simulink model "buenoensamy6"  (R2013a)
settings: Solver=ode45  StartTime=0.0  StopTime=80  FixedStep=1  RelTol=1e-3
values from neighbouring files (symbols this model uses):
  g = 9.81    [miosinlazoalgebraico1.m]    (also in proyectoy6.m)
  I1 = .004    (= 0.004)    [miosinlazoalgebraico1.m]    (also in proyectoy6.m = 0.0004)
  lc2 = .062    (= 0.062)    [miosinlazoalgebraico1.m]    (also in proyectoy6.m = 0.09)
  m2 = .7175    (= 0.7175)    [miosinlazoalgebraico1.m]    (also in proyectoy6.m = 0.0928)
  theta2 = (m2*lc2*lc2)+I2    (= 0.00775807)    [miosinlazoalgebraico1.m]    (also in proyectoy6.m = 0.00125168)
  theta3 = (m2*l1*lc2)    (= 0.008897)    [miosinlazoalgebraico1.m]    (also in proyectoy6.m = 0.00091872)
  theta4 = (m1*lc1)+(m2*l1)    (= 0.495148)    [miosinlazoalgebraico1.m]    (also in proyectoy6.m = 0.014993)
  theta5 = (m2*lc2)    (= 0.044485)    [miosinlazoalgebraico1.m]    (also in proyectoy6.m = 0.008352)
  theta6 = (m1*lc1*lc1)+(m2*l1*l1)    (= 0.09375488)    [miosinlazoalgebraico1.m]    (also in proyectoy6.m = 0.001386055)
undefined symbols (not defined in the file or in its folder): base, buenoensam, Pieza2, Pieza3, RootGround, RootPart
libraries: mblibv1 x14
settings Model: Creator=Daniel  LastModifiedBy=Daniel
settings SolverCC: MaxConsecutiveZCs=100000  ZeroCrossAlgorithm=Adaptive
settings SimMechanicsCC: VisOnUpdateDiagram=on  VisDuringSimulation=on

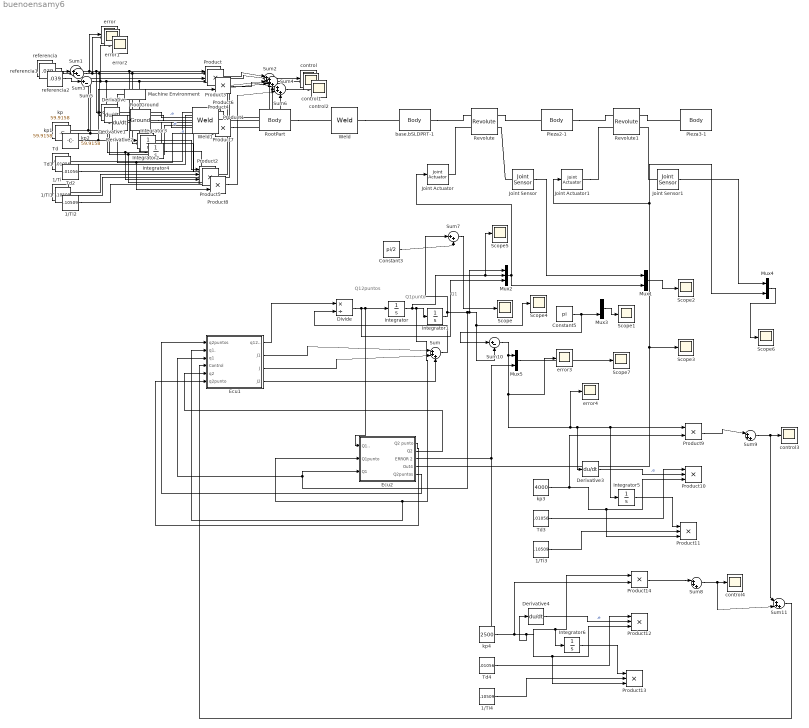
== system buenoensamy6 ==
  note: Q1
  note: Q1punto
  note: Q12puntos
  1/Ti{,1..4} (5 alike) : Constant  Value=.10509
  Constant3 : Constant  Value=pi/2
  Constant5 : Constant  Value=pi
  Derivative{,1..4} (5 alike) : Derivative
  Divide : Product  Inputs=*/
  Ecu1 : Subsystem
  Ecu2 : Subsystem
  Integrator{,2..6} (6 alike) : Integrator
  Integrator1 : Integrator  InitialCondition=pi/2  IgnoreLimit=on
  Joint Actuator : mblibv1/Sensors &  Actuators/Joint Actuator  UpdateFromCAD=off  PhysicalDomain=Mechanical  PortType=blob  ActuationStyle=Motion  AngleUnits=rad  ArcVelocityUnits=rad/s  ArcAccelerationUnits=rad/s^2  CoordPositionUnits=m  VelocityUnits=m/s  AccelerationUnits=m/s^2  ForceUnits=N  TorqueUnits=N*m  ActiveIO=on  Width=3  DialogClass=MechanicalActuatorBlock  Primitive=R1  ReferenceFrame=Absolute (World)
  Joint Actuator1 : mblibv1/Sensors &  Actuators/Joint Actuator  UpdateFromCAD=off  PhysicalDomain=Mechanical  PortType=blob  ActuationStyle=Motion  AngleUnits=rad  ArcVelocityUnits=rpm  ArcAccelerationUnits=rad/s^2  CoordPositionUnits=m  VelocityUnits=m/s  AccelerationUnits=m/s^2  ForceUnits=N  TorqueUnits=N*m  ActiveIO=on  Width=3  DialogClass=MechanicalActuatorBlock  Primitive=R1  ReferenceFrame=Absolute (World)
  Joint Sensor : mblibv1/Sensors &  Actuators/Joint Sensor  UpdateFromCAD=off  PhysicalDomain=Mechanical  PortType=blob  Muxed=on  Pose=off  Angle=on  AngleUnits=rad  ArcVelocity=off  ArcVelocityUnits=deg/s  ArcAcceleration=off  ArcAccelerationUnits=deg/s^2  CoordPosition=on  CoordPositionUnits=m  Velocity=off  VelocityUnits=m/s  Acceleration=off  AccelerationUnits=m/s^2  Quaternion=on  QuaternionDT=off  QuaternionDDT=off  QuaternionUnits=off  OutputVector=[1]  ActiveIO=on  Width=1  DialogClass=MechanicalSensorBlock  Primitive=R1  Force=off  ForceUnits=N  Torque=off  TorqueUnits=N*m  ReferenceFrame=Absolute (World)  ReactionSensedSide=Base  ReactionReferenceFrame=Absolute (World)  ReactionForce=off  ReactionForceUnits=N  ReactionMoment=off  ReactionMomentUnits=N*m
  Joint Sensor1 : mblibv1/Sensors &  Actuators/Joint Sensor  UpdateFromCAD=off  PhysicalDomain=Mechanical  PortType=blob  Muxed=on  Pose=off  Angle=on  AngleUnits=deg  ArcVelocity=off  ArcVelocityUnits=deg/s  ArcAcceleration=off  ArcAccelerationUnits=deg/s^2  CoordPosition=on  CoordPositionUnits=m  Velocity=off  VelocityUnits=m/s  Acceleration=off  AccelerationUnits=m/s^2  Quaternion=on  QuaternionDT=off  QuaternionDDT=off  QuaternionUnits=off  OutputVector=[1]  ActiveIO=on  Width=1  DialogClass=MechanicalSensorBlock  Primitive=R1  Force=off  ForceUnits=N  Torque=off  TorqueUnits=N-m  ReferenceFrame=Absolute (World)  ReactionSensedSide=Base  ReactionReferenceFrame=Absolute (World)  ReactionForce=off  ReactionForceUnits=N  ReactionMoment=off  ReactionMomentUnits=N-m
  Machine Environment : mblibv1/Bodies/Machine Environment  PortType=env  PhysicalDomain=Mechanical  DialogTemplateClass=MECH.MachineEnvironment  SyncWhenCopied=off  Gravity=[0 -9.81 0]  GravityUnits=m/s^2  GravityAsSignal=off  Dimensionality=Auto-detect  AnalysisType=Forward dynamics  LinearAssemblyTolerance=1e-3  LinearAssemblyToleranceUnits=m  AngularAssemblyTolerance=1e-3  AngularAssemblyToleranceUnits=rad  ConstraintSolverType=Stabilizing  ConstraintRelTolerance=1e-4  ConstraintAbsTolerance=1e-4  UseRobustSingularityHandling=off  RedundancyAnalysisToleranceType=Automatically select tolerance  RedundancyAnalysisTolerance=1e-14  StatePerturbationType=Fixed  PerturbationSize=1e-5  VisualizeMachine=on  BodyVisualizationType=Use model default body geometries  BodyColorSelMode=Use model default  DefaultBodyColor=[1 0 0]
  Mux{1,3..5} (4 alike) : Mux  Inputs=2
  Mux2 : Mux  Inputs=3
  Pieza2-1 : mblibv1/Bodies/Body  LConnTagsString=CS2  RConnTagsString=CS3  UpdateFromCAD=on  PMImportedID=Pieza2-1  DialogClass=MechanicalBodyBlock  Mass=0.734204  MassUnits=kg  InertiaUnits=kg*m^2  Inertia=[0.000264247,2.83059e-10,-6.28102e-08;2.83059e-10,0.0127231,5.8833e-11;-6.28102e-08,5.8833e-11,0.0126365]  Shape=Cylinder  ShapeDims=[1 1]  ShapeUnits=m  ShapeUse=false  Density=1  DensityUnits=kg/m^3  DensityUse=false  GraphicsMode=GFXFILE  GraphicsFileName=buenoensam - Pieza2-1.STL  BodyColorSelMode=COLORPALETTE  BodyColor=[1;1;0]  AttachedToCS=CS1  CG=Right$CG$[-0.0307943 -0.183465 0.38735]$WORLD$WORLD$m$[0.0349053 0 -0.999391;-0.999391 0 -0.0349053;0 1 0]$3x3 Transform$rad$WORLD$false$Pieza2-1::CG(AUTOGEN)  WorkingFrames=Right$CS1$[-0.0615922 -0.0278733 0.3683]$WORLD$WORLD$m$[0.0349053 0 -0.999391;-0.999391 0 -0.0349053;0 1 0]$3x3 Transform$rad$WORLD$false$Pieza2-1::CS1(AUTOGEN)#Left$CS2$[-0.0384461 0.0361919 0.3683]$WORLD$WORLD$m$[1 0 0;0 1 0;0 0 1]$3x3 Transform$rad$WORLD$true$Pieza2-1:-:base.bSLDPRT-1::Pieza2-1(AUTOGEN)#Right$CS3$[-0.0234804 -0.394088 0.3683]$WORLD$WORLD$m$[1 0 0;0 1 0;0 0 1]$3x3 Transform$rad$WORLD$true$Pieza2-1:-:Pieza3-1::Pieza2-1(AUTOGEN)  CGPos=[-0.0307943 -0.183465 0.38735]  CGRot=[0.0349053 0 -0.999391;-0.999391 0 -0.0349053;0 1 0]  CS0Pos=[]  CS0Rot=[]  CS1Pos=[-0.0615922 -0.0278733 0.3683]  CS1Rot=[0.0349053 0 -0.999391;-0.999391 0 -0.0349053;0 1 0]  CS2Pos=[-0.0384461 0.0361919 0.3683]  CS2Rot=[1 0 0;0 1 0;0 0 1]  CS3Pos=[-0.0234804 -0.394088 0.3683]  CS3Rot=[1 0 0;0 1 0;0 0 1]  CS4Pos=[]  CS4Rot=[]  CS5Pos=[]  CS5Rot=[]  CS6Pos=[]  CS6Rot=[]  CS7Pos=[]  CS7Rot=[]  CS8Pos=[]  CS8Rot=[]  CS9Pos=[]  CS9Rot=[]  CS10Pos=[]  CS10Rot=[]  CS11Pos=[]  CS11Rot=[]  CS12Pos=[]  CS12Rot=[]  CS13Pos=[]  CS13Rot=[]  CS14Pos=[]  CS14Rot=[]  CS15Pos=[]  CS15Rot=[]  CS16Pos=[]  CS16Rot=[]  CS17Pos=[]  CS17Rot=[]  CS18Pos=[]  CS18Rot=[]  CS19Pos=[]  CS19Rot=[]  CS20Pos=[]  CS20Rot=[]
  Pieza3-1 : mblibv1/Bodies/Body  LConnTagsString=CS2  UpdateFromCAD=on  PMImportedID=Pieza3-1  DialogClass=MechanicalBodyBlock  Mass=0.784305  MassUnits=kg  InertiaUnits=kg*m^2  Inertia=[0.000374519,0.000457935,-7.77784e-07;0.000457935,0.0141418,4.97542e-08;-7.77784e-07,4.97542e-08,0.0141799]  Shape=Cylinder  ShapeDims=[1 1]  ShapeUnits=m  ShapeUse=false  Density=1  DensityUnits=kg/m^3  DensityUse=false  GraphicsMode=GFXFILE  GraphicsFileName=buenoensam - Pieza3-1.STL  BodyColorSelMode=COLORPALETTE  BodyColor=[0;1;1]  AttachedToCS=CS1  CG=Right$CG$[-0.0137132 -0.5717 0.352532]$WORLD$WORLD$m$[0.0550174 0 -0.998485;-0.998485 0 -0.0550174;0 1 0]$3x3 Transform$rad$WORLD$false$Pieza3-1::CG(AUTOGEN)  WorkingFrames=Right$CS1$[-0.0453321 -0.458607 0.3302]$WORLD$WORLD$m$[0.0550174 0 -0.998485;-0.998485 0 -0.0550174;0 1 0]$3x3 Transform$rad$WORLD$false$Pieza3-1::CS1(AUTOGEN)#Left$CS2$[-0.0234804 -0.394088 0.3683]$WORLD$WORLD$m$[1 0 0;0 1 0;0 0 1]$3x3 Transform$rad$WORLD$true$Pieza2-1:-:Pieza3-1::Pieza3-1(AUTOGEN)  CGPos=[-0.0137132 -0.5717 0.352532]  CGRot=[0.0550174 0 -0.998485;-0.998485 0 -0.0550174;0 1 0]  CS0Pos=[]  CS0Rot=[]  CS1Pos=[-0.0453321 -0.458607 0.3302]  CS1Rot=[0.0550174 0 -0.998485;-0.998485 0 -0.0550174;0 1 0]  CS2Pos=[-0.0234804 -0.394088 0.3683]  CS2Rot=[1 0 0;0 1 0;0 0 1]  CS3Pos=[]  CS3Rot=[]  CS4Pos=[]  CS4Rot=[]  CS5Pos=[]  CS5Rot=[]  CS6Pos=[]  CS6Rot=[]  CS7Pos=[]  CS7Rot=[]  CS8Pos=[]  CS8Rot=[]  CS9Pos=[]  CS9Rot=[]  CS10Pos=[]  CS10Rot=[]  CS11Pos=[]  CS11Rot=[]  CS12Pos=[]  CS12Rot=[]  CS13Pos=[]  CS13Rot=[]  CS14Pos=[]  CS14Rot=[]  CS15Pos=[]  CS15Rot=[]  CS16Pos=[]  CS16Rot=[]  CS17Pos=[]  CS17Rot=[]  CS18Pos=[]  CS18Rot=[]  CS19Pos=[]  CS19Rot=[]  CS20Pos=[]  CS20Rot=[]
  Product{,3,6,9,14} (5 alike) : Product
  Product{1..2,4..5,7..8,10..13} (10 alike) : Product  Inputs=3
  Revolute : mblibv1/Joints/Revolute  LConnTagsString=__newl0|SA1  RConnTagsString=__newr0|SA1  UpdateFromCAD=on  PMImportedID=Pieza2-1:-:base.bSLDPRT-1  NumSAPorts=2  CutJoint=off  MarkAsCut=off  Primitives=prismatic  PrimitiveProps=R1$World$[0,0,-1]$revolute  DialogClass=JointBlock  R1Axis=[0,0,-1]
  Revolute1 : mblibv1/Joints/Revolute  LConnTagsString=__newl0|SA1  RConnTagsString=__newr0|SA1  UpdateFromCAD=on  PMImportedID=Pieza2-1:-:Pieza3-1  NumSAPorts=2  CutJoint=off  MarkAsCut=off  Primitives=prismatic  PrimitiveProps=R1$World$[0,0,1]$revolute  DialogClass=JointBlock  R1Axis=[0,0,1]
  RootGround : mblibv1/Bodies/Ground  UpdateFromCAD=on  PMImportedID=RootGround  LeftPortType=env  RightPortType=workingframe  PhysicalDomain=Mechanical  DialogClass=GroundBlock  CoordPosition=[-0.0313325,-0.14828,0.31783]  CoordPositionUnits=m  StateVectorMgrId=-1  MachineId=[0 0]  ShowEnvPort=on
  RootPart : mblibv1/Bodies/Body  LConnTagsString=CS3  RConnTagsString=CS2  UpdateFromCAD=on  PMImportedID=buenoensam/RootPart  DialogClass=MechanicalBodyBlock  Mass=0  MassUnits=kg  InertiaUnits=kg*m^2  Inertia=[0,0,0;0,0,0;0,0,0]  Shape=Cylinder  ShapeDims=[1 1]  ShapeUnits=m  ShapeUse=false  Density=1  DensityUnits=kg/m^3  DensityUse=false  GraphicsMode=MACHINE_DEFAULT  BodyColorSelMode=MACHINE_DEFAULT  BodyColor=[1;0;0]  AttachedToCS=CS1  CG=Right$CG$[-0.0313325 -0.14828 0.31783]$WORLD$WORLD$m$[1 0 0;0 1 0;0 0 1]$3x3 Transform$rad$WORLD$false$buenoensam/RootPart::CG(AUTOGEN)  WorkingFrames=Right$CS1$[0 0 0]$WORLD$WORLD$m$[1 0 0;0 1 0;0 0 1]$3x3 Transform$rad$WORLD$false$buenoensam/RootPart::CS1(AUTOGEN)#Right$CS2$[-0.0384461 0.0308496 0.278664]$WORLD$WORLD$m$[1 0 0;0 1 0;0 0 1]$3x3 Transform$rad$WORLD$true$base.bSLDPRT-1:-:buenoensam/RootPart::buenoensam/RootPart(AUTOGEN)#Left$CS3$[-0.0313325 -0.14828 0.31783]$WORLD$WORLD$m$[1 0 0;0 1 0;0 0 1]$3x3 Transform$rad$WORLD$true$RootGround:-:buenoensam/RootPart::buenoensam/RootPart(AUTOGEN)  CGPos=[-0.0313325 -0.14828 0.31783]  CGRot=[1 0 0;0 1 0;0 0 1]  CS0Pos=[]  CS0Rot=[]  CS1Pos=[0 0 0]  CS1Rot=[1 0 0;0 1 0;0 0 1]  CS2Pos=[-0.0384461 0.0308496 0.278664]  CS2Rot=[1 0 0;0 1 0;0 0 1]  CS3Pos=[-0.0313325 -0.14828 0.31783]  CS3Rot=[1 0 0;0 1 0;0 0 1]  CS4Pos=[]  CS4Rot=[]  CS5Pos=[]  CS5Rot=[]  CS6Pos=[]  CS6Rot=[]  CS7Pos=[]  CS7Rot=[]  CS8Pos=[]  CS8Rot=[]  CS9Pos=[]  CS9Rot=[]  CS10Pos=[]  CS10Rot=[]  CS11Pos=[]  CS11Rot=[]  CS12Pos=[]  CS12Rot=[]  CS13Pos=[]  CS13Rot=[]  CS14Pos=[]  CS14Rot=[]  CS15Pos=[]  CS15Rot=[]  CS16Pos=[]  CS16Rot=[]  CS17Pos=[]  CS17Rot=[]  CS18Pos=[]  CS18Rot=[]  CS19Pos=[]  CS19Rot=[]  CS20Pos=[]  CS20Rot=[]
  Scope{,1..7} (8 alike) : Scope
      Scope settings: TimeRange=15  YMin=1.5e-07  YMax=1.1e-06
      Scope1 settings: TimeRange=15  YMin=1.5707963267948  YMax=1.5707963267956  SaveName=ScopeData5
      Scope2 settings: YMin=-1.2e+17  YMax=7e+16  SaveName=ScopeData2
      Scope3 settings: YMin=-0.7  YMax=0.1  SaveName=ScopeData3
      Scope4 settings: TimeRange=15  YMin=404  YMax=424
      Scope5 settings: TimeRange=40  YMin=-0.675  YMax=-0.225  SaveName=ScopeData6
      Scope6 settings: YMin=-1.2e+17  YMax=7e+16  SaveName=ScopeData7
      Scope7 settings: YMin=-0.7  YMax=0.1  SaveName=ScopeData8
  Sum{,2,4,6,8..9,11} (7 alike) : Sum  Inputs=|+++
  Sum{1,3,5,10} (4 alike) : Sum  Inputs=|+-
  Sum7 : Sum  Inputs=|++
  Td{,1..4} (5 alike) : Constant  Value=.01056
  Weld : mblibv1/Joints/Weld  LConnTagsString=__newl0  RConnTagsString=__newr0  UpdateFromCAD=on  PMImportedID=base.bSLDPRT-1:-:buenoensam/RootPart  NumSAPorts=0  CutJoint=off  MarkAsCut=off  Primitives=weld  PrimitiveProps=W$WORLD$[0.57735,0.57735,0.57735]$weld  DialogClass=JointBlock  WAxis=[0.57735,0.57735,0.57735]
  Weld1 : mblibv1/Joints/Weld  LConnTagsString=__newl0  RConnTagsString=__newr0  UpdateFromCAD=on  PMImportedID=RootGround:-:buenoensam/RootPart  NumSAPorts=0  CutJoint=off  MarkAsCut=off  Primitives=weld  PrimitiveProps=W$WORLD$[0.57735,0.57735,0.57735]$weld  DialogClass=JointBlock  WAxis=[0.57735,0.57735,0.57735]
  base.bSLDPRT-1 : mblibv1/Bodies/Body  LConnTagsString=CS2  RConnTagsString=CS3  UpdateFromCAD=on  PMImportedID=base.bSLDPRT-1  DialogClass=MechanicalBodyBlock  Mass=1.99812  MassUnits=kg  InertiaUnits=kg*m^2  Inertia=[0.0110019,0,0;0,0.0129359,-0.000127709;0,-0.000127709,0.00347297]  Shape=Cylinder  ShapeDims=[1 1]  ShapeUnits=m  ShapeUse=false  Density=1  DensityUnits=kg/m^3  DensityUse=false  GraphicsMode=GFXFILE  GraphicsFileName=buenoensam - base.bSLDPRT-1.STL  BodyColorSelMode=COLORPALETTE  BodyColor=[0;0;1]  AttachedToCS=CS1  CG=Right$CG$[-0.0384461 0.0308496 0.278664]$WORLD$WORLD$m$[1 0 0;0 1 0;0 0 1]$3x3 Transform$rad$WORLD$false$base.bSLDPRT-1::CG(AUTOGEN)  WorkingFrames=Right$CS1$[-0.0384461 -0.00190807 0.1651]$WORLD$WORLD$m$[1 0 0;0 1 0;0 0 1]$3x3 Transform$rad$WORLD$false$base.bSLDPRT-1::CS1(AUTOGEN)#Left$CS2$[-0.0384461 0.0308496 0.278664]$WORLD$WORLD$m$[1 0 0;0 1 0;0 0 1]$3x3 Transform$rad$WORLD$true$base.bSLDPRT-1:-:buenoensam/RootPart::base.bSLDPRT-1(AUTOGEN)#Right$CS3$[-0.0384461 0.0361919 0.3683]$WORLD$WORLD$m$[1 0 0;0 1 0;0 0 1]$3x3 Transform$rad$WORLD$true$Pieza2-1:-:base.bSLDPRT-1::base.bSLDPRT-1(AUTOGEN)  CGPos=[-0.0384461 0.0308496 0.278664]  CGRot=[1 0 0;0 1 0;0 0 1]  CS0Pos=[]  CS0Rot=[]  CS1Pos=[-0.0384461 -0.00190807 0.1651]  CS1Rot=[1 0 0;0 1 0;0 0 1]  CS2Pos=[-0.0384461 0.0308496 0.278664]  CS2Rot=[1 0 0;0 1 0;0 0 1]  CS3Pos=[-0.0384461 0.0361919 0.3683]  CS3Rot=[1 0 0;0 1 0;0 0 1]  CS4Pos=[]  CS4Rot=[]  CS5Pos=[]  CS5Rot=[]  CS6Pos=[]  CS6Rot=[]  CS7Pos=[]  CS7Rot=[]  CS8Pos=[]  CS8Rot=[]  CS9Pos=[]  CS9Rot=[]  CS10Pos=[]  CS10Rot=[]  CS11Pos=[]  CS11Rot=[]  CS12Pos=[]  CS12Rot=[]  CS13Pos=[]  CS13Rot=[]  CS14Pos=[]  CS14Rot=[]  CS15Pos=[]  CS15Rot=[]  CS16Pos=[]  CS16Rot=[]  CS17Pos=[]  CS17Rot=[]  CS18Pos=[]  CS18Rot=[]  CS19Pos=[]  CS19Rot=[]  CS20Pos=[]  CS20Rot=[]
  control{,1..4} (5 alike) : Scope
      control settings: YMin=77.5  YMax=84  SaveName=ScopeData4
      control1 settings: YMin=77.5  YMax=84  SaveName=ScopeData10
      control2 settings: YMin=77.5  YMax=84  SaveName=ScopeData12
      control3 settings: YMin=77.5  YMax=84  SaveName=ScopeData14
      control4 settings: YMin=77.5  YMax=84  SaveName=ScopeData17
  error{,1..4} (5 alike) : Scope
      error settings: YMin=-0.003  YMax=0.014  SaveName=ScopeData9
      error1 settings: YMin=-0.003  YMax=0.014  SaveName=ScopeData11
      error2 settings: YMin=-0.003  YMax=0.014  SaveName=ScopeData13
      error3 settings: YMin=-0.003  YMax=0.014  SaveName=ScopeData15
      error4 settings: YMin=-0.003  YMax=0.014  SaveName=ScopeData16
  kp : Constant  Value=59.9158
  kp1 : Constant  Value=59.9158
  kp2 : Constant  Value=59.9158
  kp3 : Constant  Value=4000
  kp4 : Constant  Value=2500
  referencia : Constant  Value=.039
  referencia1 : Constant  Value=.039
  referencia2 : Constant  Value=.039
  wires:
  Divide/1 -> Mux2/3, Ecu2/1(Q1..), Integrator/1
  Integrator/1 -> Scope5/1, Mux2/2, Integrator1/1, Ecu2/2(Q1punto), Ecu1/2(q1.)
  Sum/1 -> Divide/2
  Mux2/1 -> Joint Actuator/1, Mux1/2
  Joint Sensor/1 -> Mux1/1
  Mux1/1 -> Scope2/1
  Joint Sensor1/1 -> Mux4/1
  Constant3/1 -> Sum7/2
  Sum7/1 -> Scope/1
  Constant5/1 -> Sum10/1, Mux3/2
  Ecu2/2(Q2) -> Ecu1/5("q2 ")
  Ecu2/4(Out4) -> Scope3/1, Mux4/2, Joint Actuator1/1
  Ecu2/1(Q2 punto) -> Ecu1/6(q2punto)
  Ecu1/1(q12..) -> Divide/1
  Ecu1/2(J1) -> Sum/1
  Ecu1/3(J) -> Sum/2
  Ecu1/4(J2) -> Sum/3
  Mux3/1 -> Scope1/1
  Mux4/1 -> Scope6/1
  Ecu2/5(Q2puntos) -> Ecu1/1(q2puntos)
  Mux5/1 -> Scope7/1
  Integrator1/1 -> Sum7/1, Ecu2/3("Q1 "), Ecu1/3(q1), Mux2/1, Scope4/1, Sum10/2
  referencia/1 -> Sum1/1
  Sum1/1 -> error/1, Derivative/1, Product/1, Integrator2/1
  kp/1 -> Product/2, Product2/3, Product1/3
  Product/1 -> Sum2/1
  ? -> Sum1/2
  1/Ti/1 -> Product2/2
  Product1/1 -> Sum2/3
  Sum2/1 -> control/1
  Derivative/1 -> Product1/2  ".e"
  Td/1 -> Product1/1
  Product2/1 -> Sum2/2
  Integrator2/1 -> Product2/1
  referencia1/1 -> Sum3/1
  Sum3/1 -> error1/1, Derivative1/1, Product3/1, Integrator3/1
  kp1/1 -> Product3/2, Product5/3, Product4/3
  Product3/1 -> Sum4/1
  ? -> Sum3/2
  1/Ti1/1 -> Product5/2
  Product4/1 -> Sum4/3
  Sum4/1 -> control1/1
  Derivative1/1 -> Product4/2  ".e"
  Td1/1 -> Product4/1
  Product5/1 -> Sum4/2
  Integrator3/1 -> Product5/1
  referencia2/1 -> Sum5/1
  Sum5/1 -> error2/1, Derivative2/1, Product6/1, Integrator4/1
  kp2/1 -> Product6/2, Product8/3, Product7/3
  Product6/1 -> Sum6/1
  ? -> Sum5/2
  1/Ti2/1 -> Product8/2
  Product7/1 -> Sum6/3
  Sum6/1 -> control2/1
  Derivative2/1 -> Product7/2  ".e"
  Td2/1 -> Product7/1
  Product8/1 -> Sum6/2
  Integrator4/1 -> Product8/1
  Sum10/1 -> Integrator5/1, Product9/1, Derivative3/1, error4/1, error3/1, Mux5/1
  kp3/1 -> Product10/3, Product11/3, Product9/2
  Product9/1 -> Sum9/1
  1/Ti3/1 -> Product11/2
  Sum9/1 -> Sum11/1, control3/1
  Derivative3/1 -> Product10/2  ".e"
  Td3/1 -> Product10/1
  Integrator5/1 -> Product11/1
  Ecu2/3(ERROR 2) -> Mux5/2, Product14/1, Integrator6/1, Derivative4/1
  kp4/1 -> Product14/2, Product13/3, Product12/3
  1/Ti4/1 -> Product13/2
  Sum8/1 -> Sum11/2, control4/1
  Derivative4/1 -> Product12/2  ".e"
  Td4/1 -> Product12/1
  Integrator6/1 -> Product13/1
  Product14/1 -> Sum8/1
  Sum11/1 -> Ecu1/4("Control ")
  connections:
  RootPart/RConn1 -- Weld/LConn1
  Weld/RConn1 -- base.bSLDPRT-1/LConn1
  base.bSLDPRT-1/RConn1 -- Revolute/LConn1
  Revolute/RConn1 -- Pieza2-1/LConn1
  Pieza2-1/RConn1 -- Revolute1/LConn1
  Revolute1/RConn1 -- Pieza3-1/LConn1
  RootGround/RConn1 -- Weld1/LConn1
  Weld1/RConn1 -- RootPart/LConn1
  RootGround/LConn1 -- Machine Environment/RConn1
  Joint Actuator/RConn1 -- Revolute/LConn2
  Joint Sensor/LConn1 -- Revolute/RConn2
  Joint Actuator1/RConn1 -- Revolute1/LConn2
  Joint Sensor1/LConn1 -- Revolute1/RConn2

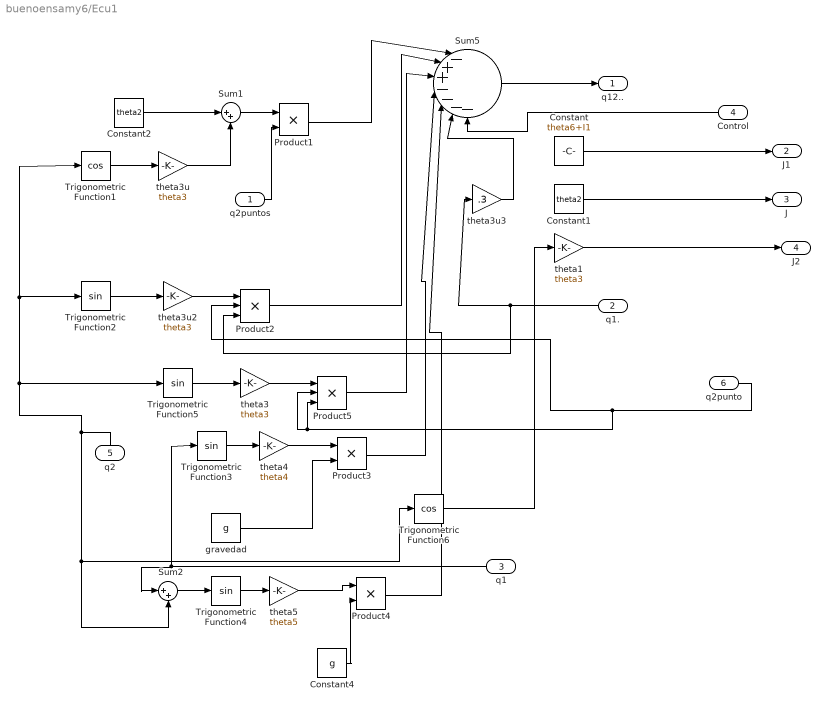
== system buenoensamy6/Ecu1 ==
  q2puntos : Inport
  q1. : Inport  Port=2
  q1 : Inport  Port=3
  "Control " : Inport  Port=4
  "q2 " : Inport  Port=5
  q2punto : Inport  Port=6
  Constant : Constant  Value=theta6+I1
  Constant1 : Constant  Value=theta2
  Constant2 : Constant  Value=theta2
  Constant4 : Constant  Value=g
  Product1 : Product
  Product2 : Product  Inputs=3
  Product3 : Product
  Product4 : Product
  Product5 : Product  Inputs=3
  Sum1 : Sum  Inputs=|++
  Sum2 : Sum  Inputs=|++
  Sum5 : Sum  Inputs=|-++----
  Trigonometric Function1 : Trigonometry  Operator=cos
  Trigonometric Function{2..5} (4 alike) : Trigonometry
  Trigonometric Function6 : Trigonometry  Operator=cos
  gravedad : Constant  Value=g
  theta1 : Gain  Gain=theta3
  "theta3 " : Gain  Gain=theta3
  theta3u : Gain  Gain=theta3
  theta3u2 : Gain  Gain=theta3
  theta3u3 : Gain  Gain=.3
  theta4 : Gain  Gain=theta4
  theta5 : Gain  Gain=theta5
  q12.. : Outport
  J1 : Outport  Port=2
  J : Outport  Port=3
  J2 : Outport  Port=4
  wires:
  Constant2/1 -> Sum1/1
  theta3u/1 -> Sum1/2
  Trigonometric Function1/1 -> theta3u/1
  Sum1/1 -> Product1/1
  q2puntos/1 -> Product1/2
  Product1/1 -> Sum5/1
  Trigonometric Function2/1 -> theta3u2/1
  theta3u2/1 -> Product2/1
  Product2/1 -> Sum5/2
  Product3/1 -> Sum5/4
  Trigonometric Function3/1 -> theta4/1
  theta4/1 -> Product3/1
  gravedad/1 -> Product3/2
  Product4/1 -> Sum5/5
  Trigonometric Function4/1 -> theta5/1
  Sum2/1 -> Trigonometric Function4/1
  theta5/1 -> Product4/1
  Constant4/1 -> Product4/2
  Constant/1 -> J1/1
  Constant1/1 -> J/1
  theta1/1 -> J2/1
  Sum5/1 -> q12../1
  "Control "/1 -> Sum5/7
  q1./1 -> Product2/3, theta3u3/1
  q1/1 -> Trigonometric Function3/1, Sum2/1
  "q2 "/1 -> Sum2/2, Trigonometric Function6/1, Trigonometric Function5/1, Trigonometric Function2/1, Trigonometric Function1/1
  q2punto/1 -> Product5/3, Product5/2, Product2/2
  Trigonometric Function5/1 -> "theta3 "/1
  "theta3 "/1 -> Product5/1
  Product5/1 -> Sum5/3
  Trigonometric Function6/1 -> theta1/1
  theta3u3/1 -> Sum5/6

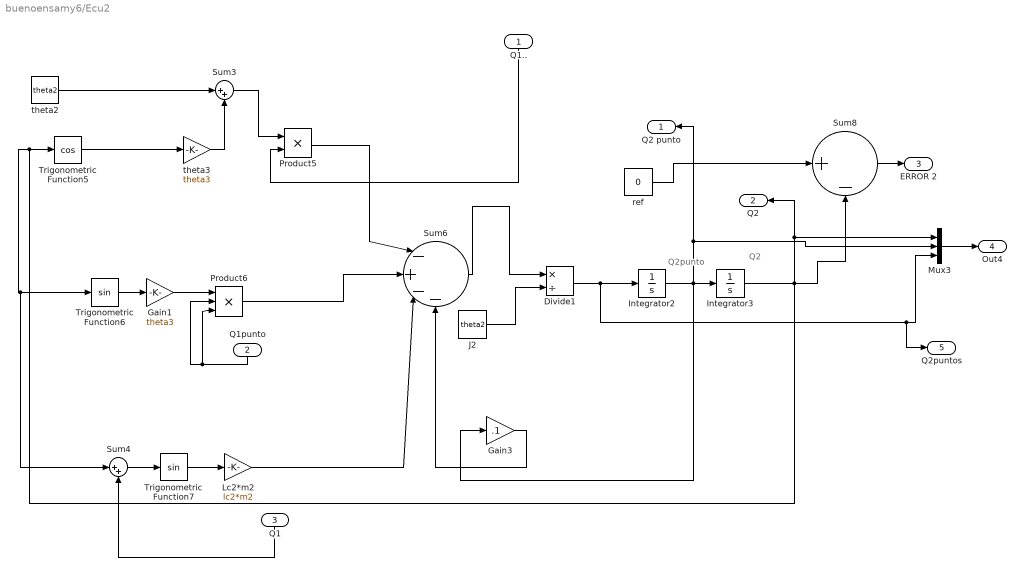
== system buenoensamy6/Ecu2 ==
  note: Q2
  note: Q2punto
  Q1.. : Inport
  Q1punto : Inport  Port=2
  "Q1 " : Inport  Port=3
  Divide1 : Product  Inputs=*/
  Gain1 : Gain  Gain=theta3
  Gain3 : Gain  Gain=.1
  Integrator2 : Integrator
  Integrator3 : Integrator
  J2 : Constant  Value=theta2
  Lc2*m2 : Gain  Gain=lc2*m2
  Mux3 : Mux  Inputs=3
  Product5 : Product
  Product6 : Product  Inputs=3
  Sum3 : Sum  Inputs=|++
  Sum4 : Sum  Inputs=|++
  Sum6 : Sum  Inputs=|-+--
  Sum8 : Sum  Inputs=|+-
  Trigonometric Function5 : Trigonometry  Operator=cos
  Trigonometric Function6 : Trigonometry
  Trigonometric Function7 : Trigonometry
  ref : Constant  Value=0
  theta2 : Constant  Value=theta2
  theta3 : Gain  Gain=theta3
  Q2 punto : Outport
  Q2 : Outport  Port=2
  ERROR 2 : Outport  Port=3
  Out4 : Outport  Port=4
  Q2puntos : Outport  Port=5
  wires:
  Trigonometric Function5/1 -> theta3/1
  theta2/1 -> Sum3/1
  theta3/1 -> Sum3/2
  Sum3/1 -> Product5/1
  Product5/1 -> Sum6/1
  Trigonometric Function6/1 -> Gain1/1
  Product6/1 -> Sum6/2
  Gain1/1 -> Product6/1
  Lc2*m2/1 -> Sum6/3
  Trigonometric Function7/1 -> Lc2*m2/1
  Sum4/1 -> Trigonometric Function7/1
  Sum6/1 -> Divide1/1
  Divide1/1 -> Q2puntos/1, Mux3/3, Integrator2/1
  J2/1 -> Divide1/2
  Integrator2/1 -> Gain3/1, Q2 punto/1, Mux3/2, Integrator3/1
  Mux3/1 -> Out4/1
  ref/1 -> Sum8/1
  Sum8/1 -> ERROR 2/1
  Integrator3/1 -> Sum4/1, Trigonometric Function6/1, Trigonometric Function5/1, Q2/1, Mux3/1, Sum8/2
  "Q1 "/1 -> Sum4/2
  Q1punto/1 -> Product6/3, Product6/2
  Q1../1 -> Product5/2
  Gain3/1 -> Sum6/4
